simulink model "lr_13"  (R2014b)
settings: Solver=ode45  StartTime=0.0  StopTime=30  RelTol=1e-3
libraries: simulink x1
settings Model: Creator=maksimka  LastModifiedBy=maksimka

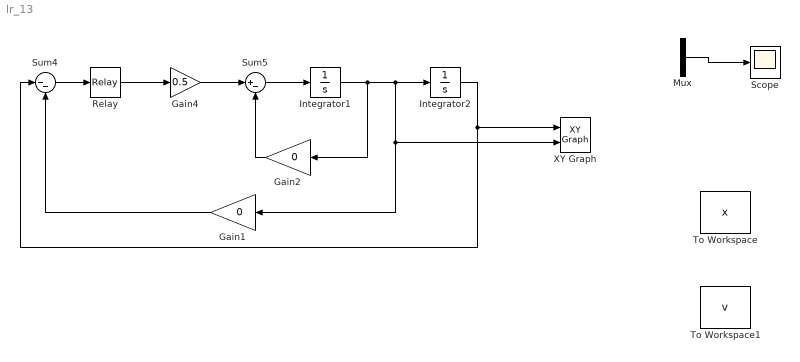
== system lr_13 ==
  Gain1 : Gain  Gain=0
  Gain2 : Gain  Gain=0
  Gain4 : Gain  Gain=0.5
  Integrator1 : Integrator
  Integrator2 : Integrator  InitialCondition=5
  Mux : Mux  Inputs=2
  Relay : Relay  OnSwitchValue=0  OffSwitchValue=0  OffOutputValue=-1
  Scope : Scope
      settings: SaveName=S13  MaxDataPoints=50000
  Sum4 : Sum  Inputs=|--
  Sum5 : Sum  Inputs=|+-
  To Workspace : ToWorkspace  VariableName=x  SampleTime=-1
      settings: Save2DSignal=2-D array (concatenate along first dimension)
  To Workspace1 : ToWorkspace  VariableName=v  SampleTime=-1
      settings: Save2DSignal=2-D array (concatenate along first dimension)
  XY Graph : simulink/Sinks/XY Graph  xmin=-10  xmax=10  ymin=-10  ymax=10  st=-1
  wires:
  Gain1/1 -> Sum4/2
  Sum4/1 -> Relay/1
  Gain4/1 -> Sum5/1
  Sum5/1 -> Integrator1/1
  Integrator2/1 -> XY Graph/1, Sum4/1
  Relay/1 -> Gain4/1
  Gain2/1 -> Sum5/2
  Mux/1 -> Scope/1
  Integrator1/1 -> Gain2/1, XY Graph/2, Gain1/1, Integrator2/1
  ? -> Mux/1
